simulink model "test"  (R2024b)
settings: Solver=VariableStepAuto  StartTime=0.0  StopTime=10.0  RelTol=1e-3
settings Model: Creator=Mehmet  LastModifiedBy=Mehmet

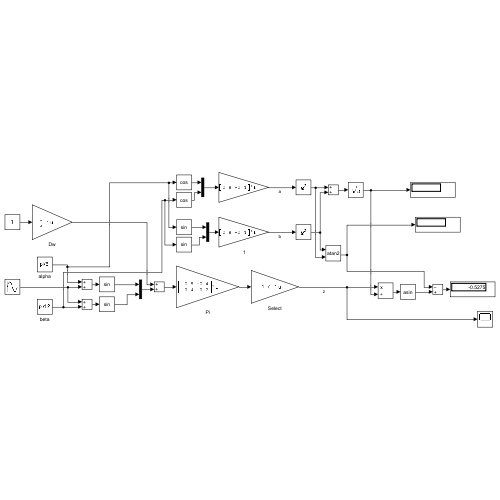
[thumbnail: Simulink's stored preview of the top-level diagram]
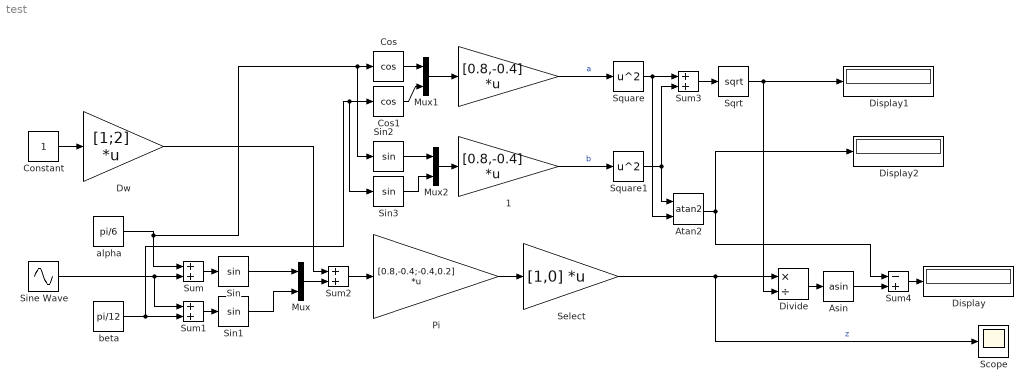
== system test ==
  " " : Gain  Gain=[0.8,-0.4]  Multiplication=Matrix(K*u)
  " 1" : Gain  Gain=[0.8,-0.4]  Multiplication=Matrix(K*u)
  Asin : Trigonometry  Operator=asin
  Atan2 : Trigonometry  Operator=atan2
  Constant : Constant
  Cos : Trigonometry  Operator=cos
  Cos1 : Trigonometry  Operator=cos
  Display : Display
  Display1 : Display
  Display2 : Display
  Divide : Product  Inputs=*/
  Dw : Gain  Gain=[1;2]  Multiplication=Matrix(K*u)
  Mux : Mux  Inputs=2
  Mux1 : Mux  Inputs=2
  Mux2 : Mux  Inputs=2
  Pi : Gain  Gain=[0.8,-0.4;-0.4,0.2]  Multiplication=Matrix(K*u)
  Scope : Scope
  Select : Gain  Gain=[1,0]  Multiplication=Matrix(K*u)
  Sin{,1..3} (4 alike) : Trigonometry
  Sine Wave : Sin  SampleTime=0
  Sqrt : Sqrt
  Square : Math  Operator=square
  Square1 : Math  Operator=square
  Sum{,1..3} (4 alike) : Sum
  Sum4 : Sum  Inputs=-+
  alpha : Constant  Value=pi/6
  beta : Constant  Value=pi/12
  wires:
  Sum/1 -> Sin/1
  alpha/1 -> Sin2/1, Cos/1, Sum/1
  Sine Wave/1 -> Sum1/1, Sum/2
  beta/1 -> Sin3/1, Cos1/1, Sum1/2
  Sum1/1 -> Sin1/1
  Sin1/1 -> Mux/2
  Sin/1 -> Mux/1
  Mux/1 -> Sum2/2
  Dw/1 -> Sum2/1
  Sum2/1 -> Pi/1
  Pi/1 -> Select/1
  Cos1/1 -> Mux1/2
  Cos/1 -> Mux1/1
  Mux1/1 -> " "/1
  Sin2/1 -> Mux2/1
  Sin3/1 -> Mux2/2
  Mux2/1 -> " 1"/1
  " "/1 -> Square/1  "a"
  " 1"/1 -> Square1/1  "b"
  Square1/1 -> Sum3/2, Atan2/1
  Square/1 -> Atan2/2, Sum3/1
  Sum3/1 -> Sqrt/1
  Select/1 -> Scope/1, Divide/1  "z"
  Sqrt/1 -> Display1/1, Divide/2
  Divide/1 -> Asin/1
  Asin/1 -> Sum4/2
  Atan2/1 -> Sum4/1, Display2/1
  Sum4/1 -> Display/1
  Constant/1 -> Dw/1
